simulink model "SimulinkPractice_02"  (R2020b)
settings: Solver=VariableStepAuto  StartTime=0.0  StopTime=10.0  RelTol=1e-3
undefined symbols (not defined in the file or in its folder): den, k, num
settings Model: Creator=riwakaram  LastModifiedBy=riwakaram

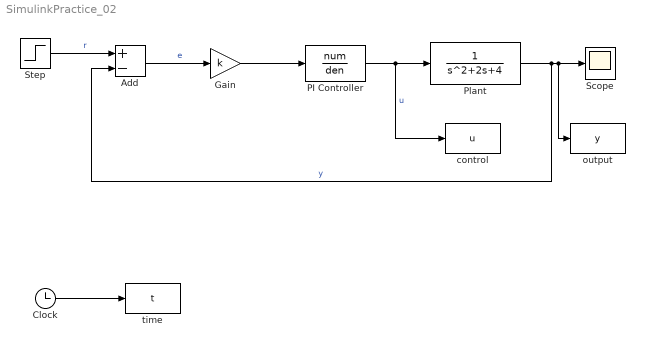
== system SimulinkPractice_02 ==
  Add : Sum  Inputs=+-
  Clock : Clock
  Gain : Gain  Gain=k
  PI Controller : TransferFcn  Numerator=num  Denominator=den
  Plant : TransferFcn  Denominator=[1 2 4]
  Scope : Scope
  Step : Step  SampleTime=0
  control : ToWorkspace  VariableName=u  SampleTime=-1
  output : ToWorkspace  VariableName=y  SampleTime=-1
  time : ToWorkspace  VariableName=t  SampleTime=-1
  wires:
  Step/1 -> Add/1  "r"
  Add/1 -> Gain/1  "e"
  Gain/1 -> PI Controller/1
  Plant/1 -> Add/2, output/1, Scope/1  "y"
  PI Controller/1 -> control/1, Plant/1  "u"
  Clock/1 -> time/1
